simulink model "State_Chart"  (R2023b)
settings: Solver=VariableStepAuto  StartTime=0.0  StopTime=10.0  RelTol=1e-3
settings Model: Creator=Eye Patch  LastModifiedBy=Eye Patch

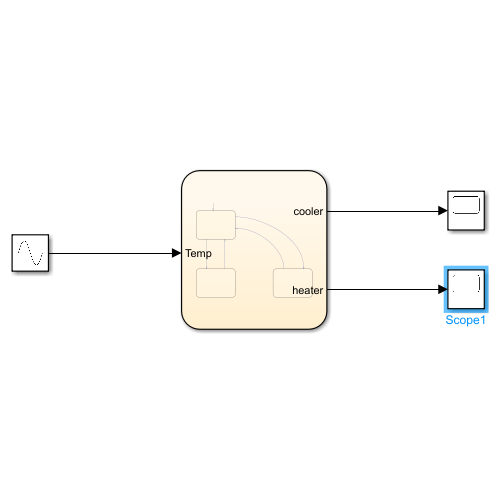
[thumbnail: Simulink's stored preview of the top-level diagram]
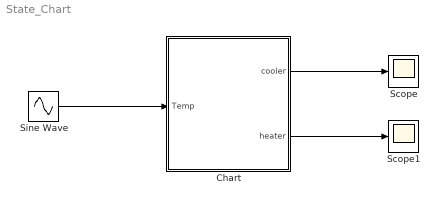
== system State_Chart ==
  Chart : Stateflow chart  TreatAsAtomicUnit=on
  Scope : Scope
  Scope1 : Scope
  Sine Wave : Sin  Amplitude=20  Bias=25  SampleTime=0
  wires:
  Chart/1(cooler) -> Scope/1
  Chart/2(heater) -> Scope1/1
  Sine Wave/1 -> Chart/1(Temp)

== stateflow chart State_Chart/Chart ==
  state First_State
    heater = 0;
    cooler = 0;
    settings: description=|
        | heater = 0;
        | cooler = 0;
  state Second_State
    heater = 1;
    cooler = 0;
    settings: description=|
        | heater = 0;
        | cooler = 0;
  state Third_State
    heater = 0;
    cooler = 1;
    settings: description=|
        | heater = 0;
        | cooler = 0;
  (default) -> First_State
  First_State -> Third_State [order 1] : [Temp > 35]
  Third_State -> First_State : [Temp<30]
  First_State -> Second_State [order 2] : [Temp < 20]
  Second_State -> First_State : [Temp > 25]
  data: Temp input; cooler output; heater output
